simulink model "MASH111"  (Simulink 8.1)
settings: Solver=FixedStepDiscrete  StartTime=0.0  StopTime=65535  FixedStep=1  RelTol=1e-3
values from neighbouring files (symbols this model uses):
  sdm_in = FRAC    (= 26625)    [PSD.m]
  w = 17    [PSD.m]
undefined symbols (not defined in the file or in its folder): qunt
libraries: simulink x1
settings Model: Creator=hazem  LastModifiedBy=amr
settings DebuggingCC: StrictBusMsg=Warning

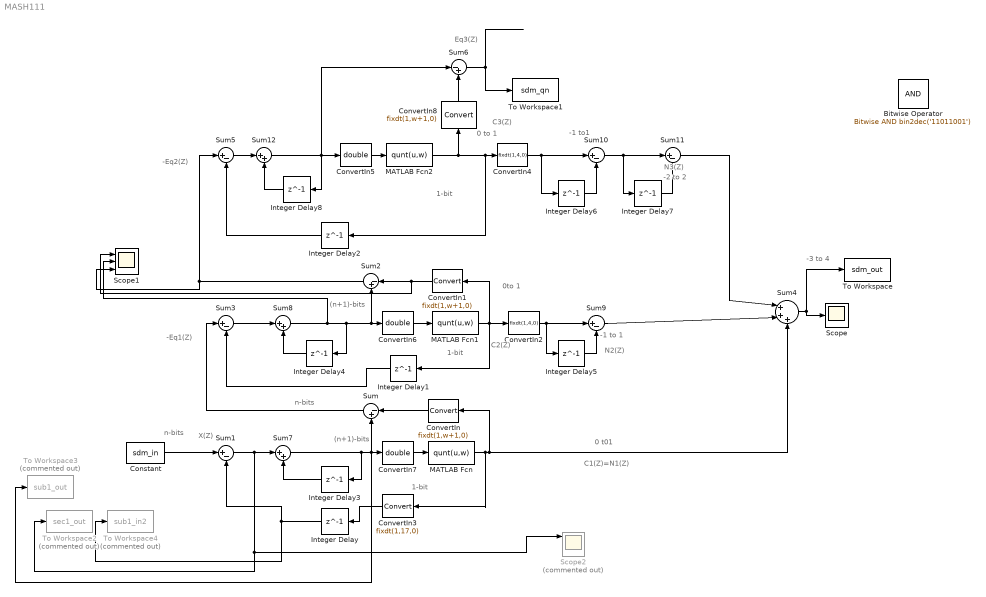
== system MASH111 ==
  note: 0 t01
  note: -1 to 1
  note: -1 to1
  note: -2 to 2
  note: 0 to 1
  note: 0to 1
  note: -3 to 4
  note: X(Z)
  note: 1-bit
  note: (n+1)-bits
  note: n-bits
  note: -Eq1(Z)
  note: C1(Z)=N1(Z)
  note: N2(Z)
  note: C2(Z)
  note: C3(Z)
  note: N3(Z)
  note: (n+1)-bits
  note: 1-bit
  note: -Eq2(Z)
  note: 1-bit
  note: n-bits
  note: Eq3(Z)
  Bitwise Operator : simulink/Logic and Bit Operations/Bitwise Operator  logicop=AND  UseBitMask=on  BitMask=bin2dec('11011001')  BitMaskRealWorld=Stored Integer
  Constant : Constant  Value=sdm_in  OutDataTypeStr=fixdt(1,w,0)
  ConvertIn : DataTypeConversion  OutDataTypeStr=fixdt(1,w+1,0)
  ConvertIn1 : DataTypeConversion  OutDataTypeStr=fixdt(1,w+1,0)
  ConvertIn2 : DataTypeConversion  OutDataTypeStr=fixdt(1,4,0)
  ConvertIn3 : DataTypeConversion  OutDataTypeStr=fixdt(1,17,0)
  ConvertIn4 : DataTypeConversion  OutDataTypeStr=fixdt(1,4,0)
  ConvertIn5 : DataTypeConversion  OutDataTypeStr=double
  ConvertIn6 : DataTypeConversion  OutDataTypeStr=double
  ConvertIn7 : DataTypeConversion  OutDataTypeStr=double
  ConvertIn8 : DataTypeConversion  OutDataTypeStr=fixdt(1,w+1,0)
  Integer Delay{,1..8} (9 alike) : Delay  DelayLength=1  InputProcessing=Inherited
  MATLAB Fcn : MATLABFcn  MATLABFcn=qunt(u,w)  OutputDimensions=1
  MATLAB Fcn1 : MATLABFcn  MATLABFcn=qunt(u,w)  OutputSignalType=real
  MATLAB Fcn2 : MATLABFcn  MATLABFcn=qunt(u,w)  OutputSignalType=real
  Scope : Scope
  Scope1 : Scope  NumInputPorts=3
      settings: YMin=-5~-5~-5  YMax=5~5~5
  Scope2 : Scope  Commented=on  NumInputPorts=3
      settings: YMin=-5~-5~-5  YMax=5~5~5  SaveName=ScopeData2
  Sum : Sum  Inputs=|-+  OutDataTypeStr=fixdt(1,w,0)  SaturateOnIntegerOverflow=on
  Sum1 : Sum  Inputs=|+-  OutDataTypeStr=fixdt(1,w,0)
  Sum10 : Sum  Inputs=|+-  OutDataTypeStr=fixdt(1,4,0)
  Sum11 : Sum  Inputs=|+-  OutDataTypeStr=fixdt(1,4,0)
  Sum12 : Sum  Inputs=|++  OutDataTypeStr=fixdt(1,w+1,0)  SaturateOnIntegerOverflow=on
  Sum2 : Sum  Inputs=|-+  OutDataTypeStr=fixdt(1,w,0)  SaturateOnIntegerOverflow=on
  Sum3 : Sum  Inputs=|+-  OutDataTypeStr=fixdt(1,w,0)
  Sum4 : Sum  Inputs=|+++  OutDataTypeStr=fixdt(1,4,0)  SaturateOnIntegerOverflow=on
  Sum5 : Sum  Inputs=|+-  OutDataTypeStr=fixdt(1,w,0)
  Sum6 : Sum  Inputs=|-+  OutDataTypeStr=fixdt(1,w,0)
  Sum7 : Sum  Inputs=|++  OutDataTypeStr=fixdt(1,w+1,0)  SaturateOnIntegerOverflow=on
  Sum8 : Sum  Inputs=|++  OutDataTypeStr=fixdt(1,w+1,0)  SaturateOnIntegerOverflow=on
  Sum9 : Sum  Inputs=|+-  OutDataTypeStr=fixdt(1,4,0)
  To Workspace : ToWorkspace  VariableName=sdm_out  SampleTime=-1
  To Workspace1 : ToWorkspace  VariableName=sdm_qn  SampleTime=-1
  To Workspace2 : ToWorkspace  Commented=on  VariableName=sec1_out  SampleTime=-1
  To Workspace3 : ToWorkspace  Commented=on  VariableName=sub1_out  SampleTime=-1
  To Workspace4 : ToWorkspace  Commented=on  VariableName=sub1_in2  SampleTime=-1
  wires:
  Sum1/1 -> Sum7/1, Scope2/1, To Workspace2/1
  MATLAB Fcn/1 -> ConvertIn3/1, Sum4/3, ConvertIn/1
  Sum3/1 -> Sum8/1
  MATLAB Fcn1/1 -> ConvertIn2/1, Integer Delay1/1, ConvertIn1/1
  Sum5/1 -> Sum12/1
  MATLAB Fcn2/1 -> ConvertIn4/1, Integer Delay2/1, ConvertIn8/1
  Sum/1 -> Sum3/1
  Sum2/1 -> Sum5/1, Scope1/3
  Sum9/1 -> Sum4/2
  Sum4/1 -> Scope/1, To Workspace/1
  Constant/1 -> Sum1/1
  Sum7/1 -> Integer Delay3/1, To Workspace3/1, ConvertIn7/1, Sum/2
  Integer Delay/1 -> Sum1/2, To Workspace4/1
  Integer Delay1/1 -> Sum3/2
  Integer Delay2/1 -> Sum5/2
  Sum11/1 -> Sum4/1
  Sum6/1 -> To Workspace1/1
  Integer Delay3/1 -> Sum7/2
  Sum8/1 -> Scope1/2, Integer Delay4/1, ConvertIn6/1, Sum2/2
  Integer Delay4/1 -> Sum8/2
  ConvertIn/1 -> Sum/1
  ConvertIn1/1 -> Scope1/1, Sum2/1
  Integer Delay5/1 -> Sum9/2
  ConvertIn2/1 -> Integer Delay5/1, Sum9/1
  ConvertIn3/1 -> Integer Delay/1
  ConvertIn4/1 -> Integer Delay6/1, Sum10/1
  Integer Delay6/1 -> Sum10/2
  Sum10/1 -> Integer Delay7/1, Sum11/1
  Integer Delay7/1 -> Sum11/2
  Integer Delay8/1 -> Sum12/2
  Sum12/1 -> Sum6/1, ConvertIn5/1, Integer Delay8/1
  ConvertIn5/1 -> MATLAB Fcn2/1
  ConvertIn6/1 -> MATLAB Fcn1/1
  ConvertIn7/1 -> MATLAB Fcn/1
  ConvertIn8/1 -> Sum6/2
